simulink model "Sim_Int_Window"  (R2021a)
settings: Solver=FixedStepAuto  StartTime=0.0  StopTime=30*TWindow  FixedStep=Ts  RelTol=1e-3
undefined symbols (not defined in the file or in its folder): N, P, Ts
settings Model: Creator=perruquetti  LastModifiedBy=perruquetti

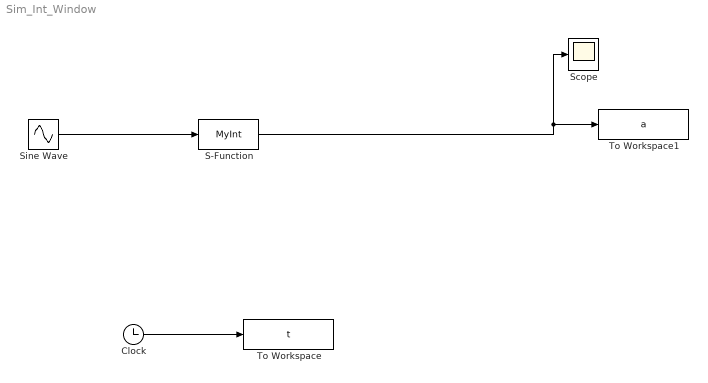
== system Sim_Int_Window ==
  Clock : Clock
  S-Function : S-Function  FunctionName=MyInt  Parameters=N,Ts,P  SFunctionDeploymentMode=off  EnableBusSupport=off
  Scope : Scope
  Sine Wave : Sin  Frequency=10  SampleTime=0
  To Workspace : ToWorkspace  VariableName=t  SampleTime=-1
  To Workspace1 : ToWorkspace  VariableName=a  SampleTime=-1
  wires:
  Clock/1 -> To Workspace/1
  S-Function/1 -> Scope/1, To Workspace1/1
  Sine Wave/1 -> S-Function/1
